simulink model "Linearization"  (R2022a)
settings: Solver=VariableStepAuto  StartTime=0.0  StopTime=100  RelTol=1e-3
undefined symbols (not defined in the file): Aactuator, ac, AeroCoeff, ControlAllocation, DUmax, DUmin, EngineTable, F, fcs, ft, g, hground, IC, kg, LandingGear, Light, LPmethod, m, MIL, Mode_deflection_aileron, Mode_deflection_elevator, Mode_deflection_rudder, Mode_deflection_TVC_y, Mode_deflection_TVC_z, N, Ninv_2nozzle, Ninv_no_nozzle, PIController, s, Sensor, slug, state0, sysID_DAQ, sysID_OBES, Umax_2nozzle, Umax_no_nozzle, Umin_2nozzle, Umin_no_nozzle, WMM2020
libraries: aerolibconvert2 x19, slpidlib x6, simulink x6, sharedutil x4, aerolibatmos2 x3, aerolibwind2 x3, aerolibbdyn x3, aerolibgravity2 x2, sharedtransform x1
(part 5 of 9)

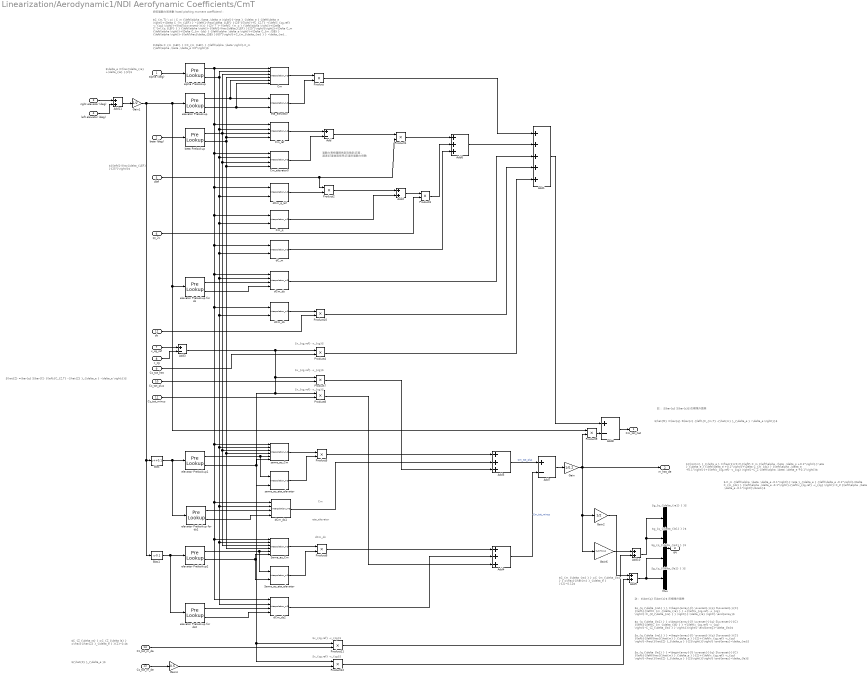
== system Linearization/Aerodynamic1/NDI Aerofynamic Coefficients/CmT ==
  note: $C_{m_{\delta_{ra} } } =C_{m_{\delta_{la} } } =\frac{{\hat{m} }_{\delta_e } }{2}∙0.12$
  note: $g_{q_{\delta_{ra1} } }$
  note: $g_{q_{\delta_{ra1} } } =\begin{array}{l} \overset{-}{q} S\overset{-}{C} {\left\{{\left(C_{m_{\delta_{ra} } } +{\left(x_{cg,ref} -x_{cg} \right)}∙C_{Z_{\delta_{ra} } } \right\}}∙\delta_{ra} \right)} \end{array}$
  note: $-C_m {\left(\alpha ,\beta ,\delta_e -0.1°\right)}{∙\eta }_{\delta_e } {\left(\delta_e -0.1°\right)}-\Delta C_{m_{ds} } {\left(\alpha ,\delta_e -0.1°\right)}-{\left(x_{cg,ref} -x_{cg} \right)}∙C_Z {\left(\alpha ,\beta ,\delta_e -0.1°\right)}\rbrack}$
  note: ${\hat{m} }_{\delta_e } =\frac{1}{0.2}{\left[\ C_m {\left(\alpha ,\beta ,\delta_e +0.1°\right)}{∙\eta }_{\delta_e } {\left(\delta_e +0.1°\right)}+\Delta C_{m_{ds} } {\left(\alpha ,\delta_e +0.1°\right)}}+{\left(x_{cg,ref} -x_{cg} \right)}∙C_Z {\left(\alpha ,\beta ,\delta_e +0.1°\right)}$
  note: $\hat{M} =\bar{q} S\bar{c} {\left\{C_{m,T} -{\hat{m} }_{\delta_e } ∙\delta_e \right\}}$
  note: dCm_ds
  note: $x_{cg,ref} -x_{cg}$
  note: eta_elevator
  note: Cm
  note: 氣動力表格僅提供到攻角到45度，
      | 超過45度後皆採用45度的氣動力係數
  note: $x_{cg,ref} -x_{cg}$
  note: $x_{cg,ref} -x_{cg}$
  note: $C_{m,T} \ =\ \ C_m {\left(\alpha ,\beta ,\delta_e \right)}{∙\eta }_{\delta_e } {\left(\delta_e \right)}+\Delta C_{m_{LEF} } ∙{\left(1-\frac{\delta_{LEF} }{25°}\right)}+C_{Z,T} ∙{\left(x_{cg,ref} -x_{cg} \right)}+\frac{q\overset{-}{c} }{2V_T }∙{\left[C_{m_q } {\left(\alpha \right)}+\Delta C_{m_{q_{LEF} } } {\left(\alpha \right)}∙{\left(1-\frac{\delta_{LEF} }{25°}\right)}\right]}+\Delta C_m {\left(\alpha \right)}+\Delta C_{m_{ds} } {\left(\alpha ,\delta_e \right)}+\Delta C_{m_{SB} } {\left(\alpha \right)}∙{\left(\frac{\delta_{SB} }{60°}\right)}+C_{m_{\delta_{ra} } } ∙\delta_{ra} +C_{m_{\delta_{la} } } ∙\delta_{la}$
  note: $\Delta C_{m_{LEF} } =C_{m_{LEF} } {\left(\alpha ,\beta \right)}-C_m {\left(\alpha ,\beta ,\delta_e =0°\right)}$
  note: 俯仰氣動力矩係數 (total pitching moment coefficient)：
  note: ${\left(1-\frac{\delta_{LEF} }{25°}\right)}$
  note: 註： $\bar{q} S\bar{c}$ 在模塊外面乘
  note: $\delta_e =\frac{\delta_{re} +\delta_{le} }{2}$
  note: $\hat{Z} =\bar{q} S\bar{C} {\left\{C_{Z,T} -{\hat{Z} }_{\delta_e } ∙\delta_e \right\}}$
  note: ${\hat{Z} }_{\delta_e }$
  note: $C_{Z_{\delta ra} } =C_{Z_{\delta la} } =\frac{{\hat{Z} }_{\delta_e } }{2}∙0.4$
  note: $g_{q_{\delta_{la1} } } =\begin{array}{l} \overset{-}{q} S\overset{-}{C} {\left\{{\left(C_{m_{\delta_{la} } } +{\left(x_{cg,ref} -x_{cg} \right)}∙C_{Z_{\delta_{la} } } \right\}}\right)} \end{array}∙\delta_{la}$
  note: $g_{q_{\delta_{re1} } } =\begin{array}{l} \overset{-}{q} S\overset{-}{C} {\left\{{\left(\frac{{\hat{m} }_{\delta_e } }{2}+{\left(x_{cg,ref} -x_{cg} \right)}∙\frac{{\hat{Z} }_{\delta_e } }{2}\right\}}\right)} \end{array}∙\delta_{re}$
  note: $g_{q_{\delta_{le1} } } =\begin{array}{l} \overset{-}{q} S\overset{-}{C} {\left\{{\left(\frac{{\hat{m} }_{\delta_e } }{2}+{\left(x_{cg,ref} -x_{cg} \right)}∙\frac{{\hat{Z} }_{\delta_e } }{2}\right\}}\right)} \end{array}∙\delta_{le}$
  note: 註： $\bar{q} S\bar{c}$ 在模塊外面乘
  note: $x_{cg,ref} -x_{cg}$
  note: $x_{cg,ref} -x_{cg}$
  note: $g_{q_{\delta_{la1} } }$
  note: $g_{q_{\delta_{re1} } }$
  note: $g_{q_{\delta_{le1} } }$
  alpha (deg) : Inport
  beta (deg) : Inport  Port=2
  right elevator (deg) : Inport  Port=3
  left elevator (deg) : Inport  Port=4
  dlef : Inport  Port=5
  qc_2v : Inport  Port=6
  x_cg_ref : Inport  Port=7
  x_cg : Inport  Port=8
  Cz_tot_hat : Inport  Port=9
  Cz_tot_plus : Inport  Port=10
  Cz_tot_minus : Inport  Port=11
  sb : Inport  Port=12
  Cz_tot_m_de : Inport  Port=13
  Cz_tot_m_da : Inport  Port=14
  Add{,3,7..8} (4 alike) : Sum  Inputs=+-
  Add1 : Sum  Inputs=+++++
  Add{2,9..11} (4 alike) : Sum
  Add4 : Sum  Inputs=+++
  Add5 : Sum  Inputs=+++
  Add6 : Sum  Inputs=+++
  Bias : Bias  Bias=+0.1  SaturateOnIntegerOverflow=off
  Bias1 : Bias  Bias=-0.1  SaturateOnIntegerOverflow=off
  Cm : Interpolation_n-D  NumberOfTableDimensions=3  Table=AeroCoeff.Cm
      settings: InputPortMap=u0,u1,u2,u3,u4,u5
  Cm_elevator0 : Interpolation_n-D  Table=AeroCoeff.Cm_elevator0
  Cm_lef : Interpolation_n-D  Table=AeroCoeff.Cm_lef
  Cm_q : Interpolation_n-D  NumberOfTableDimensions=1  Table=AeroCoeff.Cm_q
      settings: InputPortMap=u0,u1
  Gain : Gain  Gain=1/0.2
  Gain1 : Gain  Gain=1/2
  Gain2 : Gain  Gain=1/2
  Gain4 : Gain  Gain=0.5
  Gain6 : Gain  Gain=(1/2)*0.12
  Mux : Mux
  Product{,1..12} (13 alike) : Product
  Same_as_Cm : Interpolation_n-D  NumberOfTableDimensions=3  Table=AeroCoeff.Cm
      settings: InputPortMap=u0,u1,u2,u3,u4,u5
  Same_as_eta_elevator : Interpolation_n-D  NumberOfTableDimensions=1  Table=AeroCoeff.eta_elevator
      settings: InputPortMap=u0,u1
  alpha Prelookup : PreLookup  BreakpointsData=AeroCoeff.alpha_prelookup  IndexSearchMethod=Linear search  BeginIndexSearchUsingPreviousIndexResult=on  DiagnosticForOutOfRangeInput=Warning
  beta Prelookup : PreLookup  BreakpointsData=AeroCoeff.beta_prelookup  IndexSearchMethod=Linear search  BeginIndexSearchUsingPreviousIndexResult=on  DiagnosticForOutOfRangeInput=Warning
  dC_m : Interpolation_n-D  NumberOfTableDimensions=1  Table=AeroCoeff.dC_m
      settings: InputPortMap=u0,u1
  dCm_ds : Interpolation_n-D  Table=AeroCoeff.dCm_ds
  dCm_ds1 : Interpolation_n-D  Table=AeroCoeff.dCm_ds
  dCm_ds2 : Interpolation_n-D  Table=AeroCoeff.dCm_ds
  dCm_q_lef : Interpolation_n-D  NumberOfTableDimensions=1  Table=AeroCoeff.dCm_q_lef
      settings: InputPortMap=u0,u1
  dCm_sb : Interpolation_n-D  NumberOfTableDimensions=1  Table=AeroCoeff.dCm_sb
      settings: InputPortMap=u0,u1
  elevator Prelookup : PreLookup  BreakpointsData=AeroCoeff.elevator_prelookup2  IndexSearchMethod=Linear search  BeginIndexSearchUsingPreviousIndexResult=on  DiagnosticForOutOfRangeInput=Warning
  elevator Prelookup for ds : PreLookup  BreakpointsData=AeroCoeff.elevator_prelookup3  IndexSearchMethod=Linear search  BeginIndexSearchUsingPreviousIndexResult=on  DiagnosticForOutOfRangeInput=Warning
  elevator Prelookup for ds1 : PreLookup  BreakpointsData=AeroCoeff.elevator_prelookup3  IndexSearchMethod=Linear search  BeginIndexSearchUsingPreviousIndexResult=on  DiagnosticForOutOfRangeInput=Warning
  elevator Prelookup for ds2 : PreLookup  BreakpointsData=AeroCoeff.elevator_prelookup3  IndexSearchMethod=Linear search  BeginIndexSearchUsingPreviousIndexResult=on  DiagnosticForOutOfRangeInput=Warning
  elevator Prelookup1 : PreLookup  BreakpointsData=AeroCoeff.elevator_prelookup2  IndexSearchMethod=Linear search  BeginIndexSearchUsingPreviousIndexResult=on  DiagnosticForOutOfRangeInput=Warning
  elevator Prelookup2 : PreLookup  BreakpointsData=AeroCoeff.elevator_prelookup2  IndexSearchMethod=Linear search  BeginIndexSearchUsingPreviousIndexResult=on  DiagnosticForOutOfRangeInput=Warning
  eta_elevator : Interpolation_n-D  NumberOfTableDimensions=1  Table=AeroCoeff.eta_elevator
      settings: InputPortMap=u0,u1
  same_as_Cm : Interpolation_n-D  NumberOfTableDimensions=3  Table=AeroCoeff.Cm
      settings: InputPortMap=u0,u1,u2,u3,u4,u5
  same_as_eta_elevator : Interpolation_n-D  NumberOfTableDimensions=1  Table=AeroCoeff.eta_elevator
      settings: InputPortMap=u0,u1
  Cm_tot_hat : Outport  VectorParamsAs1DForOutWhenUnconnected=off
  m_hat_de : Outport  Port=2  VectorParamsAs1DForOutWhenUnconnected=off
  gq : Outport  Port=3  VectorParamsAs1DForOutWhenUnconnected=off
  wires:
  Cm/1 -> Product/1
  Cm_lef/1 -> Add/1
  Add3/1 -> Product12/1, Product11/1, Product8/1, Product7/1, Product4/1
  Product3/1 -> Add6/2
  Cm_elevator0/1 -> Add/2
  elevator Prelookup/1 -> Cm/5, eta_elevator/1
  dC_m/1 -> Add6/3
  dlef/1 -> Product2/1, Product1/2
  elevator Prelookup/2 -> Cm/6, eta_elevator/2
  right elevator (deg)/1 -> Add11/1
  Product1/1 -> Add6/1
  eta_elevator/1 -> Product/2
  beta Prelookup/2 -> Same_as_Cm/4, same_as_Cm/4, Cm_elevator0/4, Cm/4, Cm_lef/4
  Product2/1 -> Add2/1
  Cm_q/1 -> Add2/2
  beta Prelookup/1 -> Cm/3, Same_as_Cm/3, same_as_Cm/3, Cm_elevator0/3, Cm_lef/3
  Product/1 -> Add1/1
  dCm_q_lef/1 -> Product2/2
  Add2/1 -> Product3/1
  Add/1 -> Product1/1
  qc_2v/1 -> Product3/2
  alpha (deg)/1 -> alpha Prelookup/1
  Product4/1 -> Add1/5
  beta (deg)/1 -> beta Prelookup/1
  x_cg/1 -> Add3/2
  Add1/1 -> Add8/1
  Cz_tot_hat/1 -> Product4/2
  x_cg_ref/1 -> Add3/1
  Bias/1 -> elevator Prelookup for ds1/1, elevator Prelookup1/1
  Bias1/1 -> elevator Prelookup for ds2/1, elevator Prelookup2/1
  elevator Prelookup1/1 -> same_as_Cm/5, same_as_eta_elevator/1
  elevator Prelookup1/2 -> same_as_Cm/6, same_as_eta_elevator/2
  elevator Prelookup2/1 -> Same_as_eta_elevator/1, Same_as_Cm/5
  elevator Prelookup2/2 -> Same_as_Cm/6, Same_as_eta_elevator/2
  same_as_Cm/1 -> Product5/1
  same_as_eta_elevator/1 -> Product5/2
  Same_as_Cm/1 -> Product6/1
  Same_as_eta_elevator/1 -> Product6/2
  Product5/1 -> Add5/1
  Cz_tot_plus/1 -> Product7/2
  Cz_tot_minus/1 -> Product8/2
  Product7/1 -> Add5/3
  Product6/1 -> Add4/1
  Product8/1 -> Add4/3
  Add6/1 -> Add1/2
  Add5/1 -> Add7/1  "Cm_tot_plus"
  Add4/1 -> Add7/2  "Cm_tot_minus"
  Add7/1 -> Gain/1
  Product9/1 -> Add8/2
  Add8/1 -> Cm_tot_hat/1
  sb/1 -> Product10/2
  dCm_sb/1 -> Product10/1
  Product10/1 -> Add1/4
  elevator Prelookup for ds/1 -> dCm_ds/3
  elevator Prelookup for ds/2 -> dCm_ds/4
  dCm_ds/1 -> Add1/3
  elevator Prelookup for ds1/2 -> dCm_ds1/4
  elevator Prelookup for ds1/1 -> dCm_ds1/3
  alpha Prelookup/2 -> Cm/2, dCm_ds1/2, dCm_ds2/2, Same_as_Cm/2, same_as_Cm/2, dCm_sb/2, dCm_ds/2, dC_m/2, Cm_q/2, dCm_q_lef/2, Cm_elevator0/2, Cm_lef/2
  alpha Prelookup/1 -> dCm_ds1/1, dCm_ds2/1, Same_as_Cm/1, same_as_Cm/1, dCm_sb/1, dCm_ds/1, dC_m/1, Cm_q/1, dCm_q_lef/1, Cm_elevator0/1, Cm_lef/1, Cm/1
  elevator Prelookup for ds2/1 -> dCm_ds2/3
  elevator Prelookup for ds2/2 -> dCm_ds2/4
  dCm_ds1/1 -> Add5/2
  dCm_ds2/1 -> Add4/2
  Gain/1 -> m_hat_de/1, Gain2/1, Gain6/1, Product9/2
  Mux/1 -> gq/1
  Cz_tot_m_da/1 -> Product11/2
  Cz_tot_m_de/1 -> Gain4/1
  Gain2/1 -> Add9/1
  Product12/1 -> Add9/2
  Add9/1 -> Mux/4, Mux/3
  Gain6/1 -> Add10/1
  Product11/1 -> Add10/2
  Add10/1 -> Mux/1, Mux/2
  left elevator (deg)/1 -> Add11/2
  Add11/1 -> Gain1/1
  Gain1/1 -> Bias1/1, Bias/1, elevator Prelookup/1, elevator Prelookup for ds/1, Product9/1
  Gain4/1 -> Product12/2

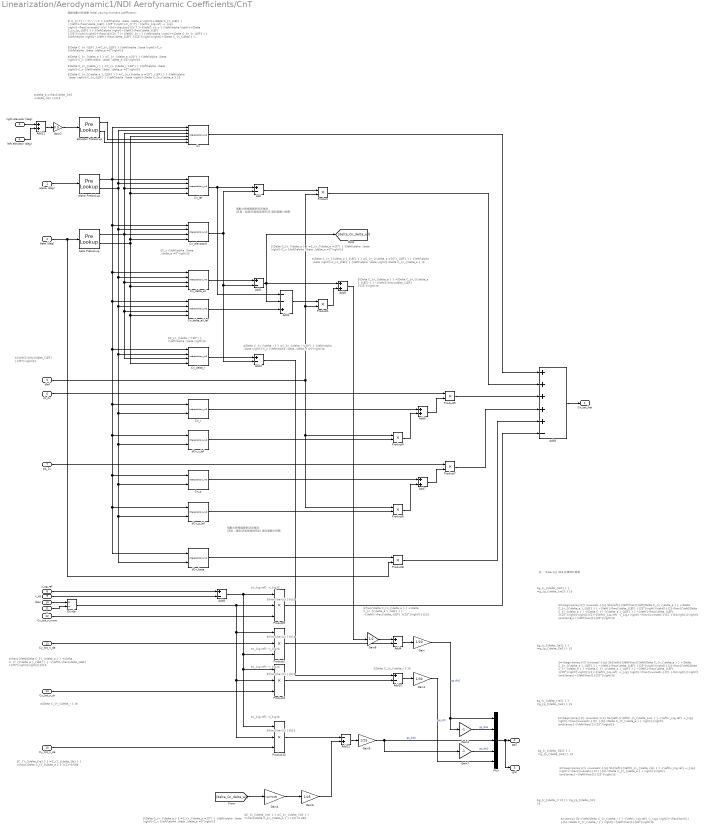
== system Linearization/Aerodynamic1/NDI Aerofynamic Coefficients/CnT ==
  note: $C_{n_{\delta_{re} } } =C_{n_{\delta_{le} } } =\frac{\Delta C_{n_{\delta_a } } }{2}∙0.26$
  note: $\Delta C_{n_{\delta_a } } +\Delta C_{n_{{\delta_a }_{LEF} } } ∙{\left(1-\frac{\delta_{LEF} }{25°}\right)}$
  note: $C_n {\left(\alpha ,\beta ,\delta_e =0°\right)}$
  note: $C_{n_{\delta_r =30°} } {\left(\alpha ,\beta \right)}$
  note: $\Delta C_{n_{\delta_r } } =C_{n_{\delta_r =30°} } {\left(\alpha ,\beta \right)}-C_n {\left(\alpha ,\beta ,\delta_e =0°\right)}$
  note: $\Delta C_{n_{\delta_r } }$
  note: $\frac{\bar{c} }{b}$
  note: $x_{cg,ref} -x_{cg}$
  note: 註： $\bar{q} Sb$ 在模塊外面乘
  note: $=\begin{array}{l} \overset{-}{q} Sb{\left\{{\left(\frac{{\left[\Delta C_{n_{\delta_a } } +\Delta C_{n_{{\delta_a }_{LEF} } } ∙{\left(1-\frac{\delta_{LEF} }{25°}\right)}\right]}}{2}-\frac{{\left[\Delta C_{Y_{\delta_a } } +\Delta C_{Y_{{\delta_a }_{LEF} } } ∙{\left(1-\frac{\delta_{LEF} }{25°}\right)}\right]}}{2}∙{\left(x_{cg,ref} -x_{cg} \right)}∙\frac{\overset{-}{C} }{b}\right\}}\right)} \end{array}∙{\left(\frac{1}{20°}\right)}$
  note: $g_{r_{\delta_{ra2} } } =g_{p_{\delta_{ra2} } }$
  note: $=\bar{q} Sb∙{\left[\Delta C_{n_{\delta_r } } -{\left(x_{cg,ref} -x_{cg} \right)}∙\frac{\bar{C} }{b}∙\Delta C_{Y_{\delta_r } } \right]}∙{\left(\frac{1}{30°}\right)}$
  note: $g_{r_{\delta_{r 2}} } =g_{p_{\delta_{r2} }$
  note: 氣動力表格僅提供到攻角到
      | 45度，超過45度後皆採用45
      | 度的氣動力係數
  note: 氣動力表格僅提供到攻角到
      | 45度，超過45度後皆採用45
      | 度的氣動力係數
  note: $x_{cg,ref} -x_{cg}$
  note: $x_{cg,ref} -x_{cg}$
  note: $\frac{\bar{c} }{b}$
  note: $\frac{\bar{c} }{b}$
  note: $\Delta C_{n_{LEF} } =C_{n_{LEF} } {\left(\alpha ,\beta \right)}-C_n {\left(\alpha ,\beta ,\delta_e =0°\right)}$
  note: 偏航氣動力矩係數 (total yawing moment coefficient)：
  note: $\Delta C_{n_{\delta_a } } =C_{n_{\delta_a =20°} } {\left(\alpha ,\beta \right)}-C_n {\left(\alpha ,\beta ,\delta_e =0°\right)}$
  note: $\Delta C_{n_{\delta_r } } =C_{n_{\delta_r =30°} } {\left(\alpha ,\beta \right)}-C_n {\left(\alpha ,\beta ,\delta_e =0°\right)}$
  note: $\Delta C_{n_{{\delta_a }_{LEF} } } =C_{n_{{\delta_a =20°}_{LEF} } } {\left(\alpha ,\beta \right)}-C_{n_{LEF} } {\left(\alpha ,\beta \right)}-\Delta C_{n_{\delta_a } }$
  note: $\ C_{n,T} \ \ =\ \ \ \ C_n {\left(\alpha ,\beta ,\delta_e \right)}+\Delta C_{n_{LEF} } ∙{\left(1-\frac{\delta_{LEF} }{25°}\right)}-C_{Y,T} ∙{\left(x_{cg,ref} -x_{cg} \right)}∙\frac{\overset{-}{c} }{b}+\frac{pb}{2V_T }∙{\left[C_{n_p } {\left(\alpha \right)}+\Delta C_{n_{p_{LEF} } } {\left(\alpha \right)}∙{\left(1-\frac{\delta_{LEF} }{25°}\right)}\right]}+\frac{rb}{2V_T }∙{\left[C_{n_r } {\left(\alpha \right)}+\Delta C_{n_{r_{LEF} } } {\left(\alpha \right)}∙{\left(1-\frac{\delta_{LEF} }{25°}\right)}\right]}+\Delta C_{n_{\beta } } {\left(\alpha \right)}∙\beta +\Delta C_{n_{\delta_r } } ∙{\left(\frac{\delta_r }{30°}\right)}+\frac{{\left[\Delta C_{n_{\delta_a } } +\Delta C_{n_{{\delta_a }_{LEF} } } ∙{\left(1-\frac{\delta_{LEF} }{25°}\right)}\right]}}{2}∙{\left(\frac{\delta_{ra} }{20°}\right)}-\frac{{\left[\Delta C_{n_{\delta_a } } +\Delta C_{n_{{\delta_a }_{LEF} } } ∙{\left(1-\frac{\delta_{LEF} }{25°}\right)}\right]}}{2}∙{\left(\frac{\delta_{la} }{20°}\right)}+C_{n_{\delta_{re} } } ∙{\left(\frac{\delta_{re} }{25°}\right)}-C_{n_{\delta_{le} } } ∙{\left(\frac{\delta_{le} }{25°}\right)}$
  note: ${\left(1-\frac{\delta_{LEF} }{25°}\right)}$
  note: $\Delta C_{n_{{\delta_a }_{LEF} } } =C_{n_{{\delta_a =20°}_{LEF} } } {\left(\alpha ,\beta \right)}-C_{n_{LEF} } {\left(\alpha ,\beta \right)}-\Delta C_{n_{\delta_a } }$
  note: $\Delta C_{n_{\delta_a } } =C_{n_{\delta_a =20°} } {\left(\alpha ,\beta \right)}-C_n {\left(\alpha ,\beta ,\delta_e =0°\right)}$
  note: $\delta_e =\frac{\delta_{re} +\delta_{le} }{2}$
  note: $\Delta C_{Y_{\delta_r } }$
  note: $\frac{{\left[\Delta C_{Y_{\delta_a } } +\Delta C_{Y_{{\delta_a }_{LEF} } } ∙{\left(1-\frac{\delta_{LEF} }{25°}\right)}\right]}}{2}$
  note: $C_{Y_{\delta_{re} } } =C_{Y_{\delta_{le} } } =\frac{\Delta C_{Y_{\delta_a } } }{2}∙0.68$
  note: $g_{r_{\delta_{la2} } } =g_{p_{\delta_{la2} } }$
  note: $=-\begin{array}{l} \overset{-}{q} Sb{\left\{{\left(\frac{{\left[\Delta C_{n_{\delta_a } } +\Delta C_{n_{{\delta_a }_{LEF} } } ∙{\left(1-\frac{\delta_{LEF} }{25°}\right)}\right]}}{2}-\frac{{\left[\Delta C_{Y_{\delta_a } } +\Delta C_{Y_{{\delta_a }_{LEF} } } ∙{\left(1-\frac{\delta_{LEF} }{25°}\right)}\right]}}{2}∙{\left(x_{cg,ref} -x_{cg} \right)}∙\frac{\overset{-}{C} }{b}\right\}}\right)} \end{array}∙{\left(\frac{1}{20°}\right)}$
  note: $g_{r_{\delta_{re2} } } =g_{p_{\delta_{re2} } }$
  note: $=\begin{array}{l} \overset{-}{q} Sb{\left\{{\left(C_{n_{\delta_{re} } } -{\left(x_{cg,ref} -x_{cg} \right)}∙\frac{\overset{-}{C} }{b}∙\Delta C_{Y_{\delta_e } } \right\}}\right)} \end{array}∙{\left(\frac{1}{25°}\right)}$
  note: $g_{r_{\delta_{le2} } } =g_{p_{\delta_{le2} } }$
  note: $=\begin{array}{l} -\overset{-}{q} Sb{\left\{{\left(C_{n_{\delta_{le} } } -{\left(x_{cg,ref} -x_{cg} \right)}∙\frac{\overset{-}{C} }{b}∙\Delta C_{Y_{\delta_e } } \right\}}\right)} \end{array}∙{\left(\frac{1}{25°}\right)}$
  note: $\frac{\Delta C_{n_{\delta_a } } +\Delta C_{n_{{\delta_a }_{LEF} } } ∙{\left(1-\frac{\delta_{LEF} }{25°}\right)}}{2}$
  note: $\Delta C_{n_{\delta_a } } =C_{n_{\delta_a =20°} } {\left(\alpha ,\beta \right)}-C_n {\left(\alpha ,\beta ,\delta_e =0°\right)}$
  note: $x_{cg,ref} -x_{cg}$
  note: $\frac{\bar{c} }{b}$
  alpha (deg) : Inport
  beta (deg) : Inport  Port=2
  right elevator (deg) : Inport  Port=3
  left elevator (deg) : Inport  Port=4
  dlef : Inport  Port=5
  rb_2v : Inport  Port=6
  pb_2v : Inport  Port=7
  x_cg_ref : Inport  Port=8
  x_cg : Inport  Port=9
  cbar : Inport  Port=10
  b : Inport  Port=11
  Cy_tot_n_mom : Inport  Port=12
  Cy_tot_n_da : Inport  Port=13
  Cy_tot_n_dr : Inport  Port=14
  Cy_tot_n_de : Inport  Port=15
  Add{,1,3..4,8,10} (6 alike) : Sum  Inputs=+-
  Add{5..7,11} (4 alike) : Sum
  Add12 : Sum  Inputs=-+
  Add2 : Sum  Inputs=--+
  Add9 : Sum  Inputs=+++++-
  Cn : Interpolation_n-D  NumberOfTableDimensions=3  Table=AeroCoeff.Cn
      settings: InputPortMap=u0,u1,u2,u3,u4,u5
  Cn_delta_ail : Interpolation_n-D  Table=AeroCoeff.Cn_delta_ail
  Cn_delta_ail_lef : Interpolation_n-D  Table=AeroCoeff.Cn_delta_ail_lef
  Cn_delta_r : Interpolation_n-D  Table=AeroCoeff.Cn_delta_r
  Cn_elevator0 : Interpolation_n-D  Table=AeroCoeff.Cn_elevator0
  Cn_lef : Interpolation_n-D  Table=AeroCoeff.Cn_lef
  Cn_p : Interpolation_n-D  NumberOfTableDimensions=1  Table=AeroCoeff.Cn_p
      settings: InputPortMap=u0,u1
  Cn_r : Interpolation_n-D  NumberOfTableDimensions=1  Table=AeroCoeff.Cn_r
      settings: InputPortMap=u0,u1
  Divide : Product  Inputs=*/
  Gain : Gain  Gain=1/20
  Gain1 : Gain  Gain=1/30
  Gain2 : Gain  Gain=0.5
  Gain3 : Gain  Gain=-1
  Gain4 : Gain  Gain=(1/2)*0.26
  Gain6 : Gain  Gain=1/25
  Gain7 : Gain  Gain=-1
  Gain8 : Gain  Gain=1/2
  Gain9 : Gain  Gain=1/25
  Mux : Mux  Inputs=5
  Product{,1,4..8} (7 alike) : Product
  Product{2..3,9..10} (4 alike) : Product  Inputs=3
  alpha Prelookup : PreLookup  BreakpointsData=AeroCoeff.alpha_prelookup  IndexSearchMethod=Linear search  BeginIndexSearchUsingPreviousIndexResult=on  DiagnosticForOutOfRangeInput=Warning
  beta Prelookup : PreLookup  BreakpointsData=AeroCoeff.beta_prelookup  IndexSearchMethod=Linear search  BeginIndexSearchUsingPreviousIndexResult=on  DiagnosticForOutOfRangeInput=Warning
  dCn_beta : Interpolation_n-D  NumberOfTableDimensions=1  Table=AeroCoeff.dCn_beta
      settings: InputPortMap=u0,u1
  dCn_p_lef : Interpolation_n-D  NumberOfTableDimensions=1  Table=AeroCoeff.dCn_p_lef
      settings: InputPortMap=u0,u1
  dCn_r_lef : Interpolation_n-D  NumberOfTableDimensions=1  Table=AeroCoeff.dCn_r_lef
      settings: InputPortMap=u0,u1
  elevator Prelookup : PreLookup  BreakpointsData=AeroCoeff.elevator_prelookup1  IndexSearchMethod=Linear search  BeginIndexSearchUsingPreviousIndexResult=on  DiagnosticForOutOfRangeInput=Warning
  Cn_tot_hat : Outport  VectorParamsAs1DForOutWhenUnconnected=off
  gp2 : Outport  Port=2  VectorParamsAs1DForOutWhenUnconnected=off
  gr2 : Outport  Port=3  VectorParamsAs1DForOutWhenUnconnected=off
  wires:
  alpha Prelookup/1 -> Cn_r/1, dCn_beta/1, dCn_p_lef/1, Cn_p/1, dCn_r_lef/1, Cn_delta_r/1, Cn_delta_ail_lef/1, Cn_delta_ail/1, Cn_elevator0/1, Cn/1, Cn_lef/1
  Add8/1 -> Product10/1, Product3/1, Product2/3, Product9/1
  Add1/1 -> Add2/2, [delta_Cn_delta_ail], Add5/1
  Cn_elevator0/1 -> Add/2, Add3/2, Add1/2
  alpha Prelookup/2 -> Cn_r/2, dCn_beta/2, dCn_p_lef/2, Cn_p/2, dCn_r_lef/2, Cn_delta_r/2, Cn_delta_ail_lef/2, Cn_delta_ail/2, Cn_elevator0/2, Cn/2, Cn_lef/2
  elevator Prelookup/1 -> Cn/5
  Add6/1 -> Product5/2
  beta Prelookup/2 -> Cn/4, Cn_lef/4, Cn_elevator0/4, Cn_delta_r/4, Cn_delta_ail_lef/4, Cn_delta_ail/4
  Cn_r/1 -> Add6/1
  Cn_delta_ail_lef/1 -> Add2/3
  pb_2v/1 -> Product7/1
  Cn_lef/1 -> Add2/1, Add/1
  Add7/1 -> Product7/2
  beta (deg)/1 -> beta Prelookup/1, Product8/2
  rb_2v/1 -> Product5/1
  Add/1 -> Product/1
  x_cg/1 -> Add8/2
  alpha (deg)/1 -> alpha Prelookup/1
  b/1 -> Divide/2
  dCn_r_lef/1 -> Product4/2
  dCn_beta/1 -> Product8/1
  Product4/1 -> Add6/2
  Divide/1 -> Product10/2, Product3/2, Product2/1, Product9/2
  x_cg_ref/1 -> Add8/1
  Cn_p/1 -> Add7/1
  dCn_p_lef/1 -> Product6/2
  Product8/1 -> Add9/5
  elevator Prelookup/2 -> Cn/6
  Cn_delta_r/1 -> Add3/1
  Product6/1 -> Add7/2
  Cy_tot_n_mom/1 -> Product9/3
  Product7/1 -> Add9/4
  Product5/1 -> Add9/3
  Add2/1 -> Product1/1
  beta Prelookup/1 -> Cn/3, Cn_lef/3, Cn_delta_r/3, Cn_delta_ail_lef/3, Cn_delta_ail/3, Cn_elevator0/3
  Cn/1 -> Add9/1
  Cn_delta_ail/1 -> Add1/1
  Add3/1 -> Add10/1
  right elevator (deg)/1 -> Add11/1
  dlef/1 -> Product4/1, Product6/1, Product/2, Product1/2
  Product/1 -> Add9/2
  Product1/1 -> Add5/2
  cbar/1 -> Divide/1
  Product9/1 -> Add9/6
  Cy_tot_n_da/1 -> Product2/2
  Product2/1 -> Add4/2
  Add5/1 -> Gain8/1
  Add4/1 -> Gain/1
  Cy_tot_n_dr/1 -> Product3/3
  Product3/1 -> Add10/2
  Add10/1 -> Gain1/1
  Add9/1 -> Cn_tot_hat/1
  Mux/1 -> gp2/1, gr2/1
  [delta_Cn_delta_ail] -> Gain4/1
  Gain3/1 -> Mux/2  "gp_dla2"
  Gain1/1 -> Mux/5  "gp_dr2"
  Gain7/1 -> Mux/4  "gp_dle2"
  Gain4/1 -> Gain6/1
  Gain6/1 -> Add12/2
  left elevator (deg)/1 -> Add11/2
  Add11/1 -> Gain2/1
  Gain2/1 -> elevator Prelookup/1
  Gain/1 -> Gain3/1, Mux/1  "gp_dla2"
  Gain8/1 -> Add4/1
  Cy_tot_n_de/1 -> Product10/3
  Product10/1 -> Add12/1
  Add12/1 -> Gain9/1
  Gain9/1 -> Mux/3, Gain7/1  "gp_dre2"

== system Linearization/Aerodynamic1/NDI Aerofynamic Coefficients/Ground Effects ==
  alpha (deg) : Inport
  beta(deg) : Inport  Port=2
  h_AGL : Inport  Port=3
  Coeff : Outport

== system Linearization/Aerodynamic1/NDI Aerofynamic Coefficients/Landing Gear Effects ==
  alpha (deg) : Inport
  beta(deg) : Inport  Port=2
  Landing Gear Angle : Inport  Port=3
  Coeff : Outport

== system Linearization/Vehicle/6DOF (Quaternion)/Accerlation_offset ==
  note: [eBook]2015 Flight vehicle system identification - a time domain methodology, Second Edition_10.8
  axyz_cg : Inport
  p : Inport  Port=2
  q : Inport  Port=3
  r : Inport  Port=4
  p_dot : Inport  Port=5
  q_dot : Inport  Port=6
  r_dot : Inport  Port=7
  position_x : Inport  Port=8
  position_y : Inport  Port=9
  position_z : Inport  Port=10
  ax_bias : Inport  Port=11
  ay_bias : Inport  Port=12
  az_bias : Inport  Port=13
  Demux : Demux  Outputs=3
  Mux : Mux  Inputs=3
  accerlation_x : Subsystem
  accerlation_y : Subsystem
  accerlation_z : Subsystem
  axyz_offset : Outport
  wires:
  az_bias/1 -> accerlation_z/10(az_bias)
  r/1 -> accerlation_x/3(r), accerlation_y/3(r), accerlation_z/5(r)
  r_dot/1 -> accerlation_y/8(r_dot), accerlation_x/6(r_dot)
  position_z/1 -> accerlation_z/4(position_z), accerlation_y/7(position_z), accerlation_x/9(position_z)
  p/1 -> accerlation_z/2(p), accerlation_y/2(p), accerlation_x/5(p)
  ay_bias/1 -> accerlation_y/10(ay_bias)
  position_y/1 -> accerlation_z/9(position_y), accerlation_y/4(position_y), accerlation_x/7(position_y)
  p_dot/1 -> accerlation_y/6(p_dot), accerlation_z/8(p_dot)
  ax_bias/1 -> accerlation_x/10(ax_bias)
  Demux/3 -> accerlation_z/1(az_cg)  "az_cg"
  position_x/1 -> accerlation_y/9(position_x), accerlation_z/7(position_x), accerlation_x/4(position_x)
  q/1 -> accerlation_x/2(q), accerlation_z/3(q), accerlation_y/5(q)
  accerlation_x/1(ax_as) -> Mux/1
  q_dot/1 -> accerlation_z/6(q_dot), accerlation_x/8(q_dot)
  Demux/2 -> accerlation_y/1(ay_cg)  "ay_cg"
  Demux/1 -> accerlation_x/1(ax_cg)  "ax_cg"
  axyz_cg/1 -> Demux/1
  accerlation_y/1(ay_as) -> Mux/2
  accerlation_z/1(az_as) -> Mux/3
  Mux/1 -> axyz_offset/1

== system Linearization/Vehicle/6DOF (Quaternion)/DCM ==
  note: ${\left[\begin{array}{c} \phi \\ \theta \\ \psi \end{array}\right]}\begin{array}{c} X\\ Y\\ Z \end{array}\to {\left[\begin{array}{c} \psi \\ \theta \\ \phi \end{array}\right]}\begin{array}{c} Z\\ Y\\ X \end{array}$
  note: $Rotation\ Order:ZYX\to \left(\psi ,\theta ,\phi \right)$
  note: ${\left[\begin{array}{c} \phi \\ \theta \\ \psi \end{array}\right]}\begin{array}{c} X\\ Y\\ Z \end{array}$
  note: 慣性座標轉至體座標的旋轉矩陣
  note: 體座標轉至慣性座標的旋轉矩陣
  Euler : Inport
  Rotation Angles to Direction Cosine Matrix : sharedtransform/Rotation Angles to Direction Cosine Matrix  rotationOrder=ZYX  aMode=aMode
      settings: SourceProductBaseCode=AE,PW,DR,MT,VE
  Selector : Selector  InputPortWidth=3  IndexOptions=Index vector (dialog)  Indices=[3 2 1]  OutputSizes=1
  Transpose : Math  Operator=transpose
  DCM_eb : Outport
  DCM_be : Outport  Port=2
  wires:
  Selector/1 -> Rotation Angles to Direction Cosine Matrix/1
  Rotation Angles to Direction Cosine Matrix/1 -> DCM_be/1, Transpose/1
  Transpose/1 -> DCM_eb/1
  Euler/1 -> Selector/1

== system Linearization/Vehicle/Actuators (no roll off)1/Engine block ==
  Mach : Inport
  Attitude : Inport  Port=2
  Add : Sum  Inputs=+-
  Add1 : Sum
  Add2 : Sum
  Constant : Constant
  Constant1 : Constant  Value=0
  Gain : Gain  Gain=64.94
  Gain1 : Gain  Gain=217.38
  If : If  IfExpression=u1<50  ElseIfExpressions=u1>=50  ShowElse=off
  If Action Subsystem : Subsystem  TreatAsAtomicUnit=on
  If Action Subsystem1 : Subsystem  TreatAsAtomicUnit=on
  If Action Subsystem2 : Subsystem  TreatAsAtomicUnit=on
  If Action Subsystem3 : Subsystem  TreatAsAtomicUnit=on
  If1 : If  IfExpression=u1<50  ElseIfExpressions=u1>=50  ShowElse=off
  Mux : Mux  Inputs=2
  Mux1 : Mux  Inputs=2
  Mux4 : Mux  Inputs=5
  Thrust Tidle : Interpolation_n-D  Table=|  InternalRulePriority=Speed
      | [1060	670	880	1140	1500	1860
      | 635	425	690	1010	1330	1700
      | 60	25	345	755	1130	1525
      | -1020	-710	-300	350	910	1360
      | -2700	-1900	-1300	-247	600	1100
      | -3600	-1400	-595	-342	-200	700]
  Thrust Tmax : Interpolation_n-D  Table=reshape([20000,21420,22700,24240,26070,28886,15000,15700,16860,18910,21075,23319,10800,11225,12250,13760,15975,18300,7000,7323,8154,9285,11115,13484,4000,4435,5000,5700,6860,8642,2500,2600,2835,3215,3950,5057],6,6)  InternalRulePriority=Speed
  Thrust Tmil : Interpolation_n-D  Table=|  InternalRulePriority=Speed
      | [12680	9150	6200	3950	2450	1400
      | 12680	9150	6313	4040	2470	1400
      | 12610	9312	6610	4290	2600	1560
      | 12640	9839	7090	4660	2840	1660
      | 12390	10176	7750	5320	3250	1930
      | 11680	9848	8050	6100	3800	2310]
  To Workspace : ToWorkspace  VariableName=T_max_min  SaveFormat=Timeseries  SampleTime=-1
  To Workspace1 : ToWorkspace  VariableName=check_engine  SaveFormat=Timeseries  SampleTime=-1
  To Workspace2 : ToWorkspace  VariableName=Mach_alt_input  SaveFormat=Timeseries  SampleTime=-1
  attitude Prelookup : PreLookup  BreakpointsData=[0,10000,20000,30000,40000,50000]  IndexSearchMethod=Linear search  BeginIndexSearchUsingPreviousIndexResult=on  DiagnosticForOutOfRangeInput=Warning
  constant : Constant  Value=117.38
  mach Prelookup : PreLookup  BreakpointsData=[0,0.2,0.4,0.6,0.8,1]  IndexSearchMethod=Linear search  BeginIndexSearchUsingPreviousIndexResult=on  DiagnosticForOutOfRangeInput=Warning
  T_max : Outport  VectorParamsAs1DForOutWhenUnconnected=off
  T_min : Outport  Port=2  VectorParamsAs1DForOutWhenUnconnected=off
  wires:
  Mach/1 -> Mux/2, mach Prelookup/1
  Attitude/1 -> attitude Prelookup/1, Mux/1
  Add2/1 -> T_min/1, Mux1/2
  Add1/1 -> T_max/1, Mux1/1
  attitude Prelookup/2 -> Thrust Tidle/4, Thrust Tmil/4, Thrust Tmax/4
  Mux1/1 -> To Workspace/1
  Thrust Tmil/1 -> Mux4/4
  Mux/1 -> To Workspace2/1
  Gain1/1 -> Add/1
  If Action Subsystem1/1(T_max1) -> Add1/2
  Constant/1 -> Gain1/1
  mach Prelookup/1 -> Thrust Tidle/1, Thrust Tmil/1, Thrust Tmax/1
  If/2 -> If Action Subsystem1/Action
  If1/2 -> If Action Subsystem3/Action
  If Action Subsystem3/1(T_min) -> Add2/2
  If Action Subsystem2/1(T_min) -> Add2/1
  If1/1 -> If Action Subsystem2/Action
  Gain/1 -> Mux4/2, If1/1
  If Action Subsystem/1(T_max1) -> Add1/1
  Thrust Tmax/1 -> Mux4/5
  mach Prelookup/2 -> Thrust Tidle/2, Thrust Tmil/2, Thrust Tmax/2
  Thrust Tidle/1 -> Mux4/3
  If/1 -> If Action Subsystem/Action
  Add/1 -> Mux4/1, If/1
  constant/1 -> Add/2
  Mux4/1 -> If Action Subsystem1/1("input "), If Action Subsystem2/1("input "), If Action Subsystem3/1("input "), To Workspace1/1, If Action Subsystem/1("input ")
  Constant1/1 -> Gain/1
  attitude Prelookup/1 -> Thrust Tidle/3, Thrust Tmil/3, Thrust Tmax/3

== system Linearization/Vehicle/Aerodynamics/Aerofynamic Coefficients ==
  note: Total Velocity
  note: 未建模，缺少數據
  note: speed brake
      | 減速板
  note: leading-edge flaps
      | 前緣襟翼
  alpha (deg) : Inport
  beta (deg) : Inport  Port=2
  right alieron (deg) : Inport  Port=3
  left aileron (deg) : Inport  Port=4
  right elevator (deg) : Inport  Port=5
  left elevator (deg) : Inport  Port=6
  rudder (deg) : Inport  Port=7
  LEF (deg) : Inport  Port=8
  SB (deg) : Inport  Port=9
  vt (ft/s) : Inport  Port=10
  p : Inport  Port=11
  q : Inport  Port=12
  r : Inport  Port=13
  GearAngle : Inport  Port=14
  h_AGL : Inport  Port=15
  Add : Sum  Inputs=+-
  CXT : Subsystem
  CYT : Subsystem
  CZT : Subsystem
  ClT : Subsystem
  CmT : Subsystem
  CnT : Subsystem
  Constant3 : Constant
  Divide2 : Product  Inputs=**/
  Divide3 : Product  Inputs=**/
  Divide4 : Product  Inputs=**/
  Gain1 : Gain  Gain=2
  Ground Effects : Subsystem  Commented=on
  Landing Gear Effects : Subsystem  Commented=on
  Terminator : Terminator  Commented=on
  Terminator1 : Terminator  Commented=on
  b(ft) : Constant  Value=ac.b
  cbar(ft) : Constant  Value=ac.cbar
  center of gravity as a fraction of cbar : Constant  Value=ac.x_cg
  r2d1 : Gain  Gain=1/25  SaturateOnIntegerOverflow=on  OutDataTypeStr=Inherit: Same as input  ParamDataTypeStr=Inherit: Same as input
  r2d3 : Gain  Gain=1/60  SaturateOnIntegerOverflow=on  OutDataTypeStr=Inherit: Same as input  ParamDataTypeStr=Inherit: Same as input
  r2d4 : Gain  Gain=1/30  SaturateOnIntegerOverflow=on  OutDataTypeStr=Inherit: Same as input  ParamDataTypeStr=Inherit: Same as input
  r2d5 : Gain  Gain=1/20  SaturateOnIntegerOverflow=on  OutDataTypeStr=Inherit: Same as input  ParamDataTypeStr=Inherit: Same as input
  r2d6 : Gain  Gain=1/20  SaturateOnIntegerOverflow=on  OutDataTypeStr=Inherit: Same as input  ParamDataTypeStr=Inherit: Same as input
  reference center of gravity as a fraction of cbar : Constant  Value=ac.x_cg_ref
  CX_T : Outport  VectorParamsAs1DForOutWhenUnconnected=off
  CY_T : Outport  Port=2  VectorParamsAs1DForOutWhenUnconnected=off
  CZ_T : Outport  Port=3  VectorParamsAs1DForOutWhenUnconnected=off
  Cl_T : Outport  Port=4  VectorParamsAs1DForOutWhenUnconnected=off
  Cm_T : Outport  Port=5  VectorParamsAs1DForOutWhenUnconnected=off
  Cn_T : Outport  Port=6  VectorParamsAs1DForOutWhenUnconnected=off
  wires:
  alpha (deg)/1 -> CnT/1(alpha (deg)), CmT/1(alpha (deg)), ClT/1(alpha (deg)), CZT/1(alpha (deg)), CYT/1(alpha (deg)), CXT/1(alpha (deg))  "alpha"
  beta (deg)/1 -> CnT/2(beta (deg)), CmT/2(beta (deg)), ClT/2(beta (deg)), CZT/2(beta (deg)), CYT/2(beta (deg)), CXT/2("beta (deg) ")  "beta"
  right elevator (deg)/1 -> CmT/9(right elevator (deg)), CnT/5("right elevator (deg) "), ClT/9(right elevator), CZT/3(right elevator (deg)), CYT/9(right elevator), CXT/3(right elevator (deg))
  vt (ft/s)/1 -> Gain1/1
  q/1 -> Divide2/1  "q"
  r/1 -> Divide3/1  "r"
  Divide2/1 -> CXT/6(qc_2v), CZT/6(qc_2v), CmT/4(qc_2v)  "qc_2v"
  Divide3/1 -> CYT/7(rb_2v), ClT/7(rb_2v), CnT/9(rb_2v)  "rb_2v"
  Divide4/1 -> CYT/8(pb_2v), ClT/8(pb_2v), CnT/10(pb_2v)  "pb_2v"
  b(ft)/1 -> CnT/14(b), Divide3/2, Divide4/2  "b"
  cbar(ft)/1 -> CnT/13(cbar), Divide2/2  "cbar"
  reference center of gravity as a fraction of cbar/1 -> CmT/5(x_cg_ref), CnT/11(x_cg_ref)
  center of gravity as a fraction of cbar/1 -> CmT/6(x_cg), CnT/12(x_cg)
  CZT/1(Cz_tot) -> CZ_T/1, CmT/7(Cz_tot)
  CYT/1(Cy_tot) -> CnT/15(Cy_tot), CY_T/1
  CXT/1(Cx_tot) -> CX_T/1
  ClT/1(Cl_tot) -> Cl_T/1
  CmT/1(Cm_tot) -> Cm_T/1
  CnT/1(Cn_tot) -> Cn_T/1
  Add/1 -> CXT/5(dlef), CnT/8(dlef), CmT/3(dlef), ClT/4(dlef), CZT/5(dlef), CYT/3(dlef)  "dlef"
  rudder (deg)/1 -> r2d4/1
  SB (deg)/1 -> r2d3/1
  r2d1/1 -> Add/2
  Constant3/1 -> Add/1
  LEF (deg)/1 -> r2d1/1
  Gain1/1 -> Divide4/3, Divide3/3, Divide2/3  "2v"
  p/1 -> Divide4/1  "p"
  r2d3/1 -> CmT/8(sb), CZT/7(sb), CXT/7(sb)
  r2d4/1 -> CYT/6(drud), CnT/7(drud), ClT/3(drud)
  GearAngle/1 -> Landing Gear Effects/3(Landing Gear Angle)
  h_AGL/1 -> Ground Effects/3(h_AGL)
  Landing Gear Effects/1(Coeff) -> Terminator/1
  Ground Effects/1(Coeff) -> Terminator1/1
  left elevator (deg)/1 -> CZT/4(left elevator (deg)), CmT/10(left elevator (deg)), CnT/6(left elevator (deg)), ClT/10(left elevator), CYT/10(left elevator), CXT/4(left elevator (deg))
  right alieron (deg)/1 -> r2d5/1
  left aileron (deg)/1 -> r2d6/1
  r2d5/1 -> CmT/11(right aileron (rad)), CnT/3(right aileron(rad)), ClT/5(right aileron(rad)), CZT/8(right aileron(rad)), CYT/4(right aileron(rad)), CXT/8(right aileron(rad))
  r2d6/1 -> CXT/9(left aileron(rad)), CZT/9(left aileron(rad)), CmT/12(left aileron (rad)), CnT/4(left aileron(rad)), ClT/6(left aileron(rad)), CYT/5(left aileron(rad))

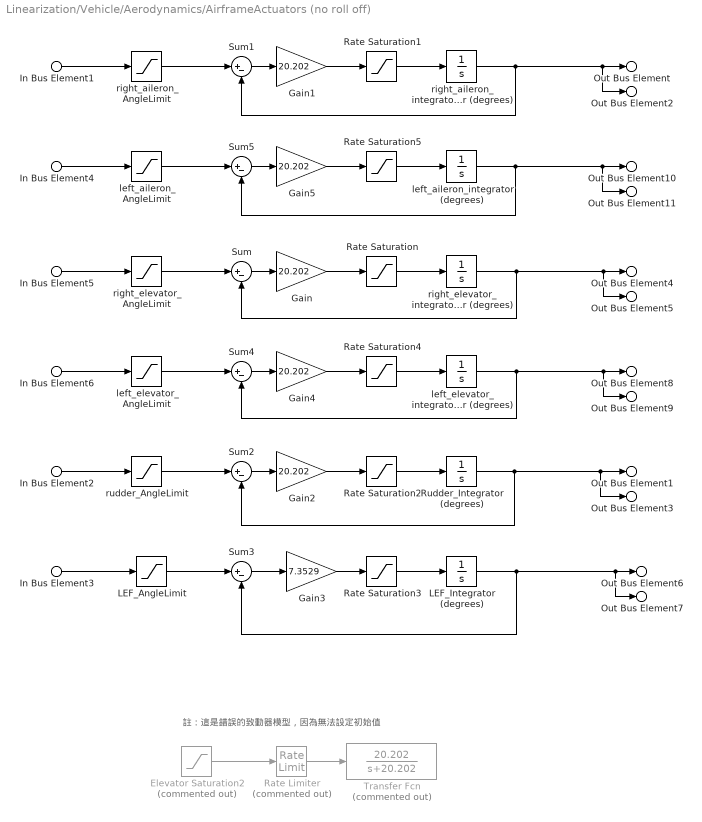
== system Linearization/Vehicle/Aerodynamics/AirframeActuators (no roll off) ==
  note: 註：這是錯誤的致動器模型，因為無法設定初始值
  In Bus Element2 : Inport  PortName=fcs_cmd  Element=rudder
  In Bus Element3 : Inport  PortName=fcs_cmd  Element=signal6
  In Bus Element4 : Inport  PortName=fcs_cmd  Element=left aileron
  In Bus Element5 : Inport  PortName=fcs_cmd  Element=right elevator
  In Bus Element6 : Inport  PortName=fcs_cmd  Element=left elevator
  In Bus Element1 : Inport  PortName=fcs_cmd  Element=right aileron
  Elevator Saturation2 : Saturate  Commented=on  UpperLimit=25  LowerLimit=-25
  Gain{,1..2,4..5} (5 alike) : Gain  Gain=20.202  SaturateOnIntegerOverflow=on  OutDataTypeStr=Inherit: Same as input  ParamDataTypeStr=Inherit: Same as input
  Gain3 : Gain  Gain=7.3529  SaturateOnIntegerOverflow=on  OutDataTypeStr=Inherit: Same as input  ParamDataTypeStr=Inherit: Same as input
  LEF_AngleLimit : Saturate  UpperLimit=Aactuator.LEF.AngleLimitUpper  LowerLimit=Aactuator.LEF.AngleLimitLower
  LEF_Integrator (degrees) : Integrator  InitialCondition=Aactuator.LEF.IntegratorInitial  LimitOutput=on  UpperSaturationLimit=Aactuator.LEF.AngleLimitUpper  LowerSaturationLimit=Aactuator.LEF.AngleLimitLower
  Rate Saturation : Saturate  UpperLimit=Aactuator.right_elevator.RateLimitUpper  LowerLimit=Aactuator.right_elevator.RateLimitLower
  Rate Saturation1 : Saturate  UpperLimit=Aactuator.right_aileron.RateLimitUpper  LowerLimit=Aactuator.right_aileron.RateLimitLower
  Rate Saturation2 : Saturate  UpperLimit=Aactuator.rudder.RateLimitUpper  LowerLimit=Aactuator.rudder.RateLimitLower
  Rate Saturation3 : Saturate  UpperLimit=Aactuator.LEF.RateLimitUpper  LowerLimit=Aactuator.LEF.RateLimitLower
  Rate Saturation4 : Saturate  UpperLimit=Aactuator.left_elevator.RateLimitUpper  LowerLimit=Aactuator.left_elevator.RateLimitLower
  Rate Saturation5 : Saturate  UpperLimit=Aactuator.left_aileron.RateLimitUpper  LowerLimit=Aactuator.left_aileron.RateLimitLower
  Rate Limiter : RateLimiter  Commented=on  RisingSlewLimit=+60  FallingSlewLimit=-60  SampleTimeMode=inherited
  Rudder_Integrator (degrees) : Integrator  InitialCondition=Aactuator.rudder.IntegratorInitial  LimitOutput=on  UpperSaturationLimit=Aactuator.rudder.AngleLimitUpper  LowerSaturationLimit=Aactuator.rudder.AngleLimitLower
  Sum{,1..5} (6 alike) : Sum  Inputs=|+-  InputSameDT=on  SaturateOnIntegerOverflow=on  OutDataTypeStr=Inherit: Same as first input
  Transfer Fcn : TransferFcn  Commented=on  Numerator=[20.202]  Denominator=[1 20.202]
  left_aileron_AngleLimit : Saturate  UpperLimit=Aactuator.left_aileron.AngleLimitUpper  LowerLimit=Aactuator.left_aileron.AngleLimitLower
  left_aileron_integrator (degrees) : Integrator  InitialCondition=Aactuator.left_aileron.IntegratorInitial  LimitOutput=on  UpperSaturationLimit=Aactuator.left_aileron.AngleLimitUpper  LowerSaturationLimit=Aactuator.left_aileron.AngleLimitLower
  left_elevator_AngleLimit : Saturate  UpperLimit=Aactuator.left_elevator.AngleLimitUpper  LowerLimit=Aactuator.left_elevator.AngleLimitLower
  left_elevator_integrator (degrees) : Integrator  InitialCondition=Aactuator.left_elevator.IntegratorInitial  LimitOutput=on  UpperSaturationLimit=Aactuator.left_elevator.AngleLimitUpper  LowerSaturationLimit=Aactuator.left_elevator.AngleLimitLower
  right_aileron_AngleLimit : Saturate  UpperLimit=Aactuator.right_aileron.AngleLimitUpper  LowerLimit=Aactuator.right_aileron.AngleLimitLower
  right_aileron_integrator (degrees) : Integrator  InitialCondition=Aactuator.right_aileron.IntegratorInitial  LimitOutput=on  UpperSaturationLimit=Aactuator.right_aileron.AngleLimitUpper  LowerSaturationLimit=Aactuator.right_aileron.AngleLimitLower
  right_elevator_AngleLimit : Saturate  UpperLimit=Aactuator.right_elevator.AngleLimitUpper  LowerLimit=Aactuator.right_elevator.AngleLimitLower  LinearizeAsGain=off
  right_elevator_integrator (degrees) : Integrator  InitialCondition=Aactuator.right_elevator.IntegratorInitial  LimitOutput=on  UpperSaturationLimit=Aactuator.right_elevator.AngleLimitUpper  LowerSaturationLimit=Aactuator.right_elevator.AngleLimitLower
  rudder_AngleLimit : Saturate  UpperLimit=Aactuator.rudder.AngleLimitUpper  LowerLimit=Aactuator.rudder.AngleLimitLower
  Out Bus Element : Outport  PortName=ActPositions  Element=right Aileron_deg
  Out Bus Element1 : Outport  PortName=ActPositions  Element=Rudder_deg
  Out Bus Element4 : Outport  PortName=ActPositions  Element=right Elevator_deg
  Out Bus Element6 : Outport  PortName=ActPositions  Element=LEF_deg
  Out Bus Element8 : Outport  PortName=ActPositions  Element=left Elevator_deg
  Out Bus Element10 : Outport  PortName=ActPositions  Element=left Aileron_deg
  Out Bus Element2 : Outport  Port=2  PortName=ActSensor_Out  Element=right Aileron_deg
  Out Bus Element3 : Outport  Port=2  PortName=ActSensor_Out  Element=Rudder_deg
  Out Bus Element5 : Outport  Port=2  PortName=ActSensor_Out  Element=right Elevator_deg
  Out Bus Element7 : Outport  Port=2  PortName=ActSensor_Out  Element=LEF_deg
  Out Bus Element9 : Outport  Port=2  PortName=ActSensor_Out  Element=left Elevator_deg
  Out Bus Element11 : Outport  Port=2  PortName=ActSensor_Out  Element=left Aileron_deg
  wires:
  Gain/1 -> Rate Saturation/1
  Gain1/1 -> Rate Saturation1/1
  In Bus Element5/1 -> right_elevator_AngleLimit/1
  Rate Saturation/1 -> right_elevator_integrator (degrees)/1
  right_aileron_integrator (degrees)/1 -> Out Bus Element2/1, Out Bus Element/1, Sum1/2
  Rate Saturation1/1 -> right_aileron_integrator (degrees)/1
  Gain2/1 -> Rate Saturation2/1
  Sum1/1 -> Gain1/1
  Rudder_Integrator (degrees)/1 -> Out Bus Element3/1, Out Bus Element1/1, Sum2/2
  Rate Saturation2/1 -> Rudder_Integrator (degrees)/1
  Sum/1 -> Gain/1
  Sum2/1 -> Gain2/1
  right_elevator_integrator (degrees)/1 -> Sum/2, Out Bus Element5/1, Out Bus Element4/1
  In Bus Element1/1 -> right_aileron_AngleLimit/1
  In Bus Element2/1 -> rudder_AngleLimit/1
  LEF_Integrator (degrees)/1 -> Out Bus Element6/1, Out Bus Element7/1, Sum3/2
  In Bus Element3/1 -> LEF_AngleLimit/1
  Sum3/1 -> Gain3/1
  Rate Saturation3/1 -> LEF_Integrator (degrees)/1
  Gain3/1 -> Rate Saturation3/1
  Sum4/1 -> Gain4/1
  Gain4/1 -> Rate Saturation4/1
  Rate Saturation4/1 -> left_elevator_integrator (degrees)/1
  In Bus Element6/1 -> left_elevator_AngleLimit/1
  left_elevator_integrator (degrees)/1 -> Sum4/2, Out Bus Element9/1, Out Bus Element8/1
  Gain5/1 -> Rate Saturation5/1
  Rate Saturation5/1 -> left_aileron_integrator (degrees)/1
  Sum5/1 -> Gain5/1
  left_aileron_integrator (degrees)/1 -> Out Bus Element11/1, Out Bus Element10/1, Sum5/2
  In Bus Element4/1 -> left_aileron_AngleLimit/1
  right_aileron_AngleLimit/1 -> Sum1/1
  left_aileron_AngleLimit/1 -> Sum5/1
  left_elevator_AngleLimit/1 -> Sum4/1
  right_elevator_AngleLimit/1 -> Sum/1
  rudder_AngleLimit/1 -> Sum2/1
  LEF_AngleLimit/1 -> Sum3/1
  Rate Limiter/1 -> Transfer Fcn/1
  Elevator Saturation2/1 -> Rate Limiter/1

== system Linearization/Vehicle/Aerodynamics/Leading Edge Flap ==
  note: $\delta_{LEF} =1.38\frac{2s+7.25}{s+7.25}\alpha -9.05\frac{\bar{q} }{p_s }+1.45$
      | $\alpha$ 的單位：deg
      | $\bar{q}$ 是動壓， $p_s$ 是靜壓，兩者單位要一致 (公制：1Pa = 1 $N/m^2$ = 1 $\mathrm{kg}/\left(m{\cdot s}^2 \right)$ ；英制：1psf = 1 $\mathrm{lbf}/{\mathrm{ft}}^2$ = 1 $\mathrm{slugs}/\left(\mathrm{ft}\cdot s^2 \right)$ )
  vt (m/s) : Inport
  rho (kg/m^3) : Inport  Port=2
  P (Pa) : Inport  Port=3
  alpha (deg) : Inport  Port=4
  Divide1 : Product  Inputs=*/
  Divide2 : Product  Inputs=**
  Gain2 : Gain  Gain=1.38  SaturateOnIntegerOverflow=on  OutDataTypeStr=Inherit: Same as input  ParamDataTypeStr=Inherit: Same as input
  LEF Rate Limiter : RateLimiter  RisingSlewLimit=Aactuator.LEF.RateLimitUpper  FallingSlewLimit=Aactuator.LEF.RateLimitLower  SampleTimeMode=inherited  InitialCondition=Aactuator.LEF.IntegratorInitial
  LEF Saturation : Saturate  UpperLimit=Aactuator.LEF.AngleLimitUpper  LowerLimit=Aactuator.LEF.AngleLimitLower
  Square1 : Math  Operator=square  SignedPower=on
  Sum : Sum  Inputs=-|+|+  InputSameDT=on  SaturateOnIntegerOverflow=on  OutDataTypeStr=Inherit: Same as first input
  Transfer Fcn : TransferFcn  Numerator=[2 7.25]  Denominator=[1 7.25]
  coeff1 : Constant  Value=1.45
  r2d2 : Gain  Gain=0.5  SaturateOnIntegerOverflow=on  OutDataTypeStr=Inherit: Same as input  ParamDataTypeStr=Inherit: Same as input
  r2d6 : Gain  Gain=9.05  SaturateOnIntegerOverflow=on  OutDataTypeStr=Inherit: Same as input  ParamDataTypeStr=Inherit: Same as input
  Out Bus Element3 : Outport  PortName=ActSensor_Out  Element=LEF_deg
  Out Bus Element2 : Outport  Port=2  PortName=ActPositions  Element=LEF_deg
  wires:
  Transfer Fcn/1 -> Gain2/1
  coeff1/1 -> Sum/3
  r2d6/1 -> Sum/1
  Square1/1 -> Divide2/1
  alpha (deg)/1 -> Transfer Fcn/1  "alpha (deg)"
  P (Pa)/1 -> Divide1/2
  vt (m/s)/1 -> Square1/1
  rho (kg/m^3)/1 -> Divide2/2  "rho(kg/m^3)"
  Divide1/1 -> r2d6/1
  Sum/1 -> LEF Saturation/1
  LEF Saturation/1 -> LEF Rate Limiter/1
  Divide2/1 -> r2d2/1
  r2d2/1 -> Divide1/1  "qbar (Pa)"
  Gain2/1 -> Sum/2
  LEF Rate Limiter/1 -> Out Bus Element2/1, Out Bus Element3/1

== system Linearization/Vehicle/LandingGear GroundReaction/L Main Gear Geometry Forces and Moments ==
  note: $z_c^E$
  note: $z_g^E$
  note: 飛機重心在慣性座標的高度
  note: 詹庭宇:
      | 此起落架模組源自MATLAB Simulink Example:HL-20
      | 我有做正負號的訂正
  note: 詹庭宇:
      | 此起落架模組源自MATLAB Simulink Example:HL-20
      | 我有做正負號的訂正
  note: 定義：
      | 慣性座標+Z軸朝下
      | 體座標+Z軸朝下
  note: $z_g^E =z_c^E +C_{31} {\left(x_g^b -x_c^b \right)}+C_{32} {\left(y_g^b -y_c^b \right)}+C_{33} {\left(z_g^b -z_c^b \right)}$
  note: $z_r^E$
  note: 體座標轉至慣性座標的旋轉矩陣
  note: 體座標轉至慣性座標的旋轉矩陣
  note: 詹庭宇:拿掉/忽略輪胎側向力模型，Fy=0
  ground_z_ft : Inport
  plant : Inport  Port=2
  GearLoc : Inport  Port=3
  Bus Selector3 : BusSelector  OutputSignals=altitude,DCM_eb,DCM_be
  Calc Gear Force and Pos : Subsystem
  GenerateGroundFM : Subsystem
  Rotate pos to earth axes : Product  Multiplication=Matrix(*)  InputSameDT=on  SaturateOnIntegerOverflow=on  OutDataTypeStr=Inherit: Same as first input
  Sum3 : Sum
  Zg : Selector  InputPortWidth=3  IndexOptions=Index vector (dialog)  Indices=3  OutputSizes=1
  detect_WOW : RelationalOperator  OutDataTypeStr=boolean  InputSameDT=off
  FM : Outport
  WOW : Outport  Port=2
  GearCmprs : Outport  Port=3
  wires:
  Rotate pos to earth axes/1 -> Zg/1
  Bus Selector3/1 -> [ZcL], [Xe]  "<altitude>"
  detect_WOW/1 -> GenerateGroundFM/Enable, WOW/1, Calc Gear Force and Pos/1(WOW)
  Bus Selector3/2 -> [DCM_eb]  "<DCM_eb>"
  Zg/1 -> Sum3/2
  Sum3/1 -> detect_WOW/1
  Calc Gear Force and Pos/3(ZgB_prime) -> GenerateGroundFM/3(ZgB_prime)
  GearLoc/1 -> Calc Gear Force and Pos/3(Xg), Rotate pos to earth axes/2, GenerateGroundFM/1(GearLoc)
  Calc Gear Force and Pos/1(dZ_strut) -> GearCmprs/1
  [DCM_eb] -> Calc Gear Force and Pos/5(DCM_eb)
  GenerateGroundFM/1(FM) -> FM/1
  [Xe] -> Sum3/1
  [DCM_eb] -> Rotate pos to earth axes/1
  Calc Gear Force and Pos/2(Fn_strut) -> GenerateGroundFM/2(Fn_strut)
  plant/1 -> Bus Selector3/1, GenerateGroundFM/5(plant)
  ground_z_ft/1 -> detect_WOW/2, Calc Gear Force and Pos/2(ZrL)
  Bus Selector3/3 -> GenerateGroundFM/4(DCM_be)  "<DCM_be>"
  [ZcL] -> Calc Gear Force and Pos/4(ZcL)

== system Linearization/Vehicle/LandingGear GroundReaction/Nose Gear Geometry Forces and Moments ==
  note: $z_c^E$
  note: $z_g^E$
  note: 飛機重心在慣性座標的高度
  note: 詹庭宇:
      | 此起落架模組源自MATLAB Simulink Example:HL-20
      | 我有做正負號的訂正
  note: 詹庭宇:
      | 此起落架模組源自MATLAB Simulink Example:HL-20
      | 我有做正負號的訂正
  note: 定義：
      | 慣性座標+Z軸朝下
      | 體座標+Z軸朝下
  note: $z_g^E =z_c^E +C_{31} {\left(x_g^b -x_c^b \right)}+C_{32} {\left(y_g^b -y_c^b \right)}+C_{33} {\left(z_g^b -z_c^b \right)}$
  note: $z_r^E$
  note: 體座標轉至慣性座標的旋轉矩陣
  note: 體座標轉至慣性座標的旋轉矩陣
  note: 詹庭宇:拿掉/忽略輪胎側向力模型，Fy=0
  ground_z_ft : Inport
  plant : Inport  Port=2
  GearLoc : Inport  Port=3
  Bus Selector3 : BusSelector  OutputSignals=altitude,DCM_eb,DCM_be
  Calc Gear Force and Pos : Subsystem
  GenerateGroundFM : Subsystem
  Rotate pos to earth axes : Product  Multiplication=Matrix(*)  InputSameDT=on  SaturateOnIntegerOverflow=on  OutDataTypeStr=Inherit: Same as first input
  Sum3 : Sum
  Zg : Selector  InputPortWidth=3  IndexOptions=Index vector (dialog)  Indices=3  OutputSizes=1
  detect_WOW : RelationalOperator  OutDataTypeStr=boolean  InputSameDT=off
  FM : Outport
  WOW : Outport  Port=2
  GearCmprs : Outport  Port=3
  wires:
  Rotate pos to earth axes/1 -> Zg/1
  Bus Selector3/1 -> [ZcL], [Xe]  "<altitude>"
  detect_WOW/1 -> GenerateGroundFM/Enable, WOW/1, Calc Gear Force and Pos/1(WOW)
  Zg/1 -> Sum3/2
  Sum3/1 -> detect_WOW/1
  Calc Gear Force and Pos/3(ZgB_prime) -> GenerateGroundFM/3(ZgB_prime)
  GearLoc/1 -> GenerateGroundFM/1(GearLoc), Calc Gear Force and Pos/3(Xg), Rotate pos to earth axes/2
  Calc Gear Force and Pos/1(dZ_strut) -> GearCmprs/1
  [DCM_eb] -> Calc Gear Force and Pos/5(DCM_eb)
  GenerateGroundFM/1(FM) -> FM/1
  [Xe] -> Sum3/1
  [DCM_eb] -> Rotate pos to earth axes/1
  Calc Gear Force and Pos/2(Fn_strut) -> GenerateGroundFM/2(Fn_strut)
  plant/1 -> Bus Selector3/1, GenerateGroundFM/5(plant)
  ground_z_ft/1 -> detect_WOW/2, Calc Gear Force and Pos/2(ZrL)
  [ZcL] -> Calc Gear Force and Pos/4(ZcL)
  Bus Selector3/2 -> [DCM_eb]  "<DCM_eb>"
  Bus Selector3/3 -> GenerateGroundFM/4(DCM_be)  "<DCM_be>"

== system Linearization/Vehicle/LandingGear GroundReaction/R Main Gear Geometry Forces and Moments ==
  note: $z_c^E$
  note: $z_g^E$
  note: 飛機重心在慣性座標的高度
  note: 詹庭宇:
      | 此起落架模組源自MATLAB Simulink Example:HL-20
      | 我有做正負號的訂正
  note: 詹庭宇:
      | 此起落架模組源自MATLAB Simulink Example:HL-20
      | 我有做正負號的訂正
  note: 定義：
      | 慣性座標+Z軸朝下
      | 體座標+Z軸朝下
  note: $z_g^E =z_c^E +C_{31} {\left(x_g^b -x_c^b \right)}+C_{32} {\left(y_g^b -y_c^b \right)}+C_{33} {\left(z_g^b -z_c^b \right)}$
  note: $z_r^E$
  note: 體座標轉至慣性座標的旋轉矩陣
  note: 體座標轉至慣性座標的旋轉矩陣
  note: 詹庭宇:拿掉/忽略輪胎側向力模型，Fy=0
  ground_z_ft : Inport
  plant : Inport  Port=2
  GearLoc : Inport  Port=3
  Bus Selector3 : BusSelector  OutputSignals=altitude,DCM_eb,DCM_be
  Calc Gear Force and Pos : Subsystem
  GenerateGroundFM : Subsystem
  Rotate pos to earth axes : Product  Multiplication=Matrix(*)  InputSameDT=on  SaturateOnIntegerOverflow=on  OutDataTypeStr=Inherit: Same as first input
  Sum3 : Sum
  Zg : Selector  InputPortWidth=3  IndexOptions=Index vector (dialog)  Indices=3  OutputSizes=1
  detect_WOW : RelationalOperator  OutDataTypeStr=boolean  InputSameDT=off
  FM : Outport
  WOW : Outport  Port=2
  GearCmprs : Outport  Port=3
  wires:
  Rotate pos to earth axes/1 -> Zg/1
  Bus Selector3/1 -> [ZcL], [Xe]  "<altitude>"
  detect_WOW/1 -> Calc Gear Force and Pos/1(WOW), GenerateGroundFM/Enable, WOW/1
  Zg/1 -> Sum3/2
  Sum3/1 -> detect_WOW/1
  Calc Gear Force and Pos/3(ZgB_prime) -> GenerateGroundFM/3(ZgB_prime)
  GearLoc/1 -> Rotate pos to earth axes/2, GenerateGroundFM/1(GearLoc), Calc Gear Force and Pos/3(Xg)
  Calc Gear Force and Pos/1(dZ_strut) -> GearCmprs/1
  [DCM_eb] -> Calc Gear Force and Pos/5(DCM_eb)
  GenerateGroundFM/1(FM) -> FM/1
  [Xe] -> Sum3/1
  [DCM_eb] -> Rotate pos to earth axes/1
  Calc Gear Force and Pos/2(Fn_strut) -> GenerateGroundFM/2(Fn_strut)
  plant/1 -> GenerateGroundFM/5(plant), Bus Selector3/1
  ground_z_ft/1 -> detect_WOW/2, Calc Gear Force and Pos/2(ZrL)
  [ZcL] -> Calc Gear Force and Pos/4(ZcL)
  Bus Selector3/2 -> [DCM_eb]  "<DCM_eb>"
  Bus Selector3/3 -> GenerateGroundFM/4(DCM_be)  "<DCM_be>"
